simulink model "envolventeContenedores"  (R2021a)
settings: Solver=VariableStepAuto  StartTime=0.0  StopTime=10.0  RelTol=1e-3
values from neighbouring files (symbols this model uses):
  estado_cont = [x_positions; hy_cont]    [perfilObsaculos.m]    (also in valoresPlanta_29_9_24.m = [x_positions; [hy_muelle hy_cont]])
settings Model: Creator=agustin  LastModifiedBy=agustin

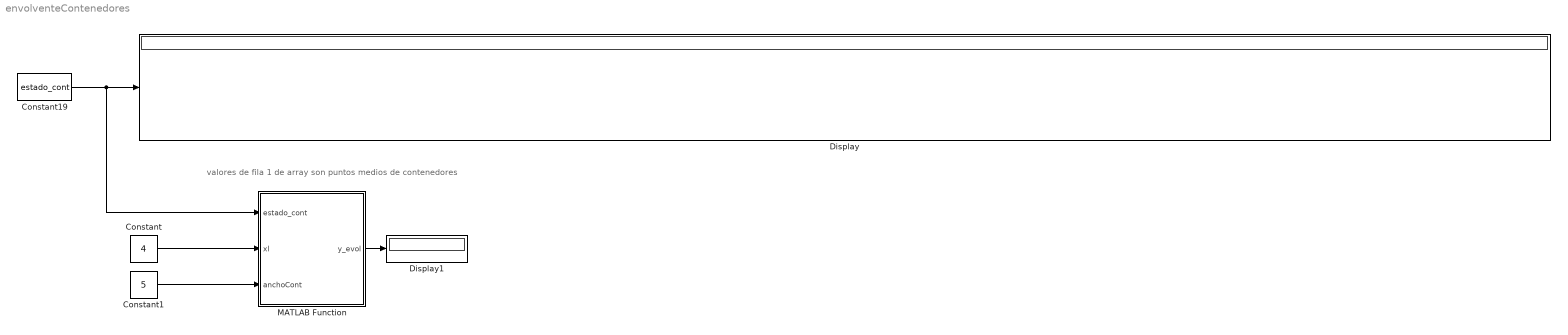
== system envolventeContenedores ==
  note: valores de fila 1 de array son puntos medios de contenedores
  Constant : Constant  Value=4
  Constant1 : Constant  Value=5
  Constant19 : Constant  Value=estado_cont
  Display : Display
  Display1 : Display
  MATLAB Function : MATLAB Function  TreatAsAtomicUnit=on
  wires:
  Constant19/1 -> MATLAB Function/1(estado_cont), Display/1
  Constant/1 -> MATLAB Function/2(xl)
  Constant1/1 -> MATLAB Function/3(anchoCont)
  MATLAB Function/1(y_evol) -> Display1/1

== matlab function envolventeContenedores/MATLAB Function ==
  data: estado_cont input; y_evol output; xl input; anchoCont input
function y_evol = envolvente(estado_cont, xl, anchoCont)
%Calculo de envolvente. Hay un perfil de contenedores. 
%Se debe usar la posicion actual de la carga para comparar con la altura
%que debe tener el contenedor (teniendo en cuenta el indice del vector)
%si la carga esta entre los limites del contenedor(i) (contenedor(i) -
%contenedor(i)aX*0.5 y contenedor(i) + contenedor(i)aX*0.5)
% Dividir la posicion en x de la carga por el ancho de contenedores para
% obtener la posicion del indice  (usar floor?) --> si da 0 por ejemplo la
% la altura del envolvente sera igual a la del contenedor en el indice 0
% mas el factor de seguridad. Para el modo de contacto no usar el factor de
% seguridad.
fseg = 2.5;
index = floor(xl/anchoCont)+1;
%si xl es menor a 0 (con las posiciones corregidas, sin el offset,
%modificar los valores para que sean 0 (muelle) o la altura de un camion
if (index<0)
    y_evol = 0+fseg; %por ahora solo muelle

elseif (index>=0 && index<=20)
    y_evol = estado_cont(2,index) + fseg;
elseif (index>20)
    %no deberia pasar 
    y_evol = -5+fseg;
else
    y_evol = 0;
end
end
